simulink model "sadycos"  (R2024b)
settings: Solver=VariableStepAuto  StartTime=0.0  StopTime=60  RelTol=1e-3
undefined symbols (not defined in the file): BusTemplates, Parameters
settings Model: Creator=Friedrich Tuttas  LastModifiedBy=fn103921
settings DebuggingCC: AllowedUnitSystems=SI,SI (extended)
settings RTWCC: GPUComputeCapability=3.5

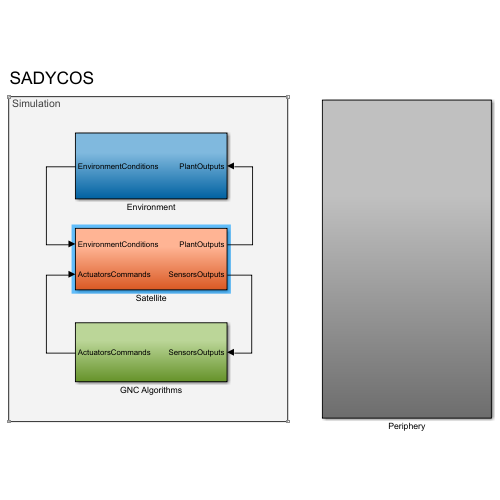
[thumbnail: Simulink's stored preview of the top-level diagram]
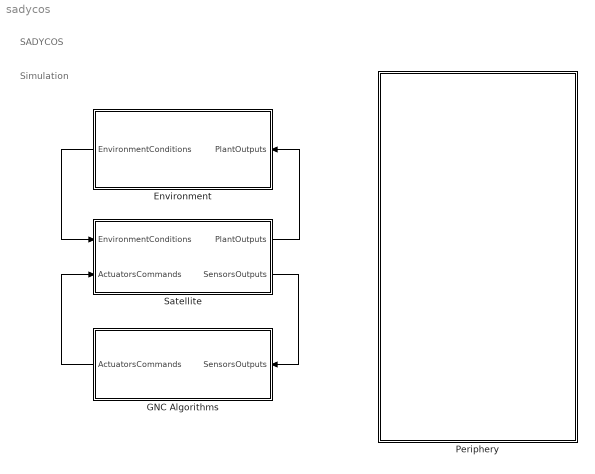
== system sadycos ==
  note: SADYCOS
  note: Simulation
  Environment : Subsystem
  GNC Algorithms : Subsystem
  Periphery : Subsystem
  Satellite : Subsystem
  wires:
  Satellite/1(PlantOutputs) -> Environment/1(PlantOutputs)
  Satellite/2(SensorsOutputs) -> GNC Algorithms/1(SensorsOutputs)
  GNC Algorithms/1(ActuatorsCommands) -> Satellite/2(ActuatorsCommands)
  Environment/1(EnvironmentConditions) -> Satellite/1(EnvironmentConditions)

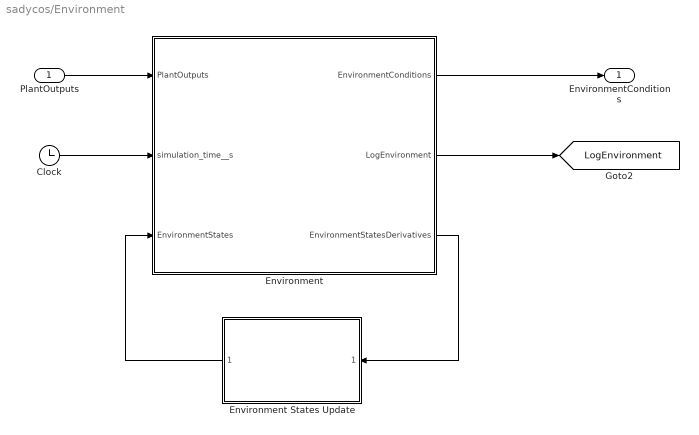
== system sadycos/Environment ==
  PlantOutputs : Inport
  Clock : Clock
  Environment : MATLAB Function  TreatAsAtomicUnit=on  SystemSampleTime=[0 0]
  Environment States Update : Subsystem  ReferencedSubsystem=states_update  states_type=Parameters.General.States.Type.Environment  bus=EnvironmentStates  BusTemplate=BusTemplates.EnvironmentStates  BusInitialValue=Parameters.General.States.InitialStates.Environment
  EnvironmentConditions : Outport
  tag scope: LogEnvironment=global
  wires:
  PlantOutputs/1 -> Environment/1(PlantOutputs)
  Clock/1 -> Environment/2(simulation_time__s)
  Environment/1(EnvironmentConditions) -> EnvironmentConditions/1
  Environment/3(EnvironmentStatesDerivatives) -> Environment States Update/1
  Environment/2(LogEnvironment) -> [LogEnvironment]
  Environment States Update/1 -> Environment/3(EnvironmentStates)

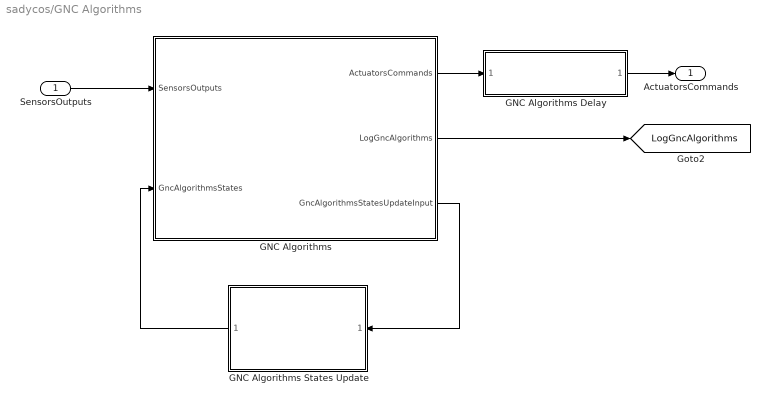
== system sadycos/GNC Algorithms ==
  SensorsOutputs : Inport
  GNC Algorithms : MATLAB Function  TreatAsAtomicUnit=on  SystemSampleTime=Parameters.General.SampleTimeParameters__s.GncAlgorithms
  GNC Algorithms Delay : Subsystem  ReferencedSubsystem=delay  delay_type=Parameters.General.Delays.Type.GncAlgorithms  delay_value=Parameters.General.Delays.Value.GncAlgorithms  bus=ActuatorsCommands  BusTemplate=BusTemplates.ActuatorsCommands  BusInitialValue=Parameters.General.Delays.InitialOutputs.GncAlgorithms
  GNC Algorithms States Update : Subsystem  ReferencedSubsystem=states_update  states_type=Parameters.General.States.Type.GncAlgorithms  bus=GncAlgorithmsStates  BusTemplate=BusTemplates.GncAlgorithmsStates  BusInitialValue=Parameters.General.States.InitialStates.GncAlgorithms
  ActuatorsCommands : Outport
  tag scope: LogGncAlgorithms=global
  wires:
  SensorsOutputs/1 -> GNC Algorithms/1(SensorsOutputs)
  GNC Algorithms States Update/1 -> GNC Algorithms/2(GncAlgorithmsStates)
  GNC Algorithms/3(GncAlgorithmsStatesUpdateInput) -> GNC Algorithms States Update/1
  GNC Algorithms/1(ActuatorsCommands) -> GNC Algorithms Delay/1
  GNC Algorithms Delay/1 -> ActuatorsCommands/1
  GNC Algorithms/2(LogGncAlgorithms) -> [LogGncAlgorithms]

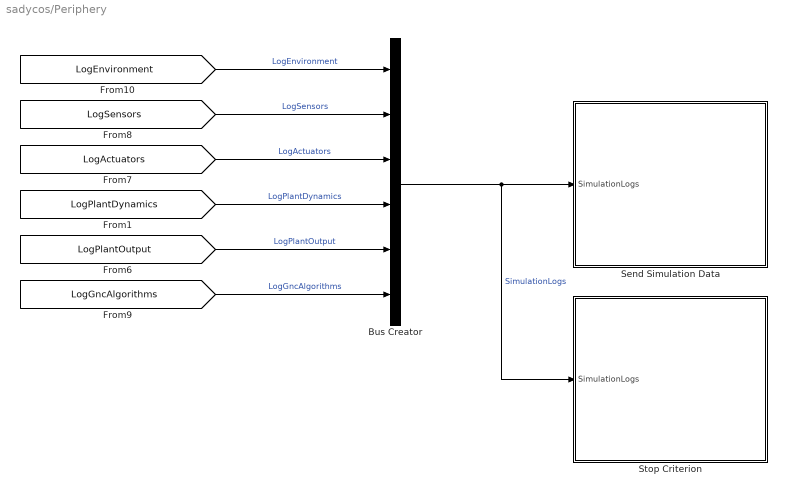
== system sadycos/Periphery ==
  Bus Creator : BusCreator  Inputs=6
  Send Simulation Data : Subsystem  Variant=on
  Stop Criterion : Subsystem  Variant=on
  wires:
  [LogEnvironment] -> Bus Creator/1  "LogEnvironment"
  [LogSensors] -> Bus Creator/2  "LogSensors"
  [LogActuators] -> Bus Creator/3  "LogActuators"
  [LogPlantDynamics] -> Bus Creator/4  "LogPlantDynamics"
  [LogGncAlgorithms] -> Bus Creator/6  "LogGncAlgorithms"
  Bus Creator/1 -> Stop Criterion/1(SimulationLogs), Send Simulation Data/1(SimulationLogs)  "SimulationLogs"
  [LogPlantOutput] -> Bus Creator/5  "LogPlantOutput"

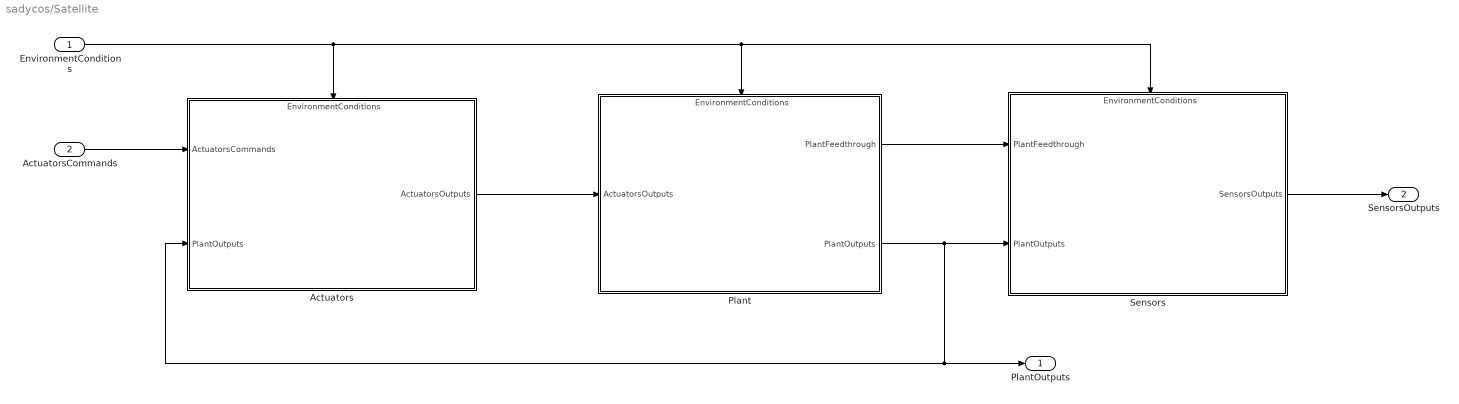
== system sadycos/Satellite ==
  EnvironmentConditions : Inport
  ActuatorsCommands : Inport  Port=2
  Actuators : Subsystem
      settings: PortSchema="{\"entries\":[{\"content\":{\"sides\":[{\"content\":{\"connectorIds\":[\"In1\",\"In2\"]},\"type\":\"ConnectorPlacement.EquallySpacedRectSide\",\"uuid\":\"84ab0471-c988-440c-b8b5-169cbd29501d\"},{\"content\":{\"connectorIds\":[\"Out1\"],\"side\":\"RIGHT\"},\"type\":\"ConnectorPlacement.EquallySpacedRectSide\",\"uuid\":\"27e08eb0-e385-4cd2-ab07-f71ebf995a80\"},{\"content\":{\"connectorIds\":[\"In3\"],\"side\":\"TOP\"},\"type\":\"ConnectorPlacement.EquallySpacedRectSide\",\"uuid\":\"cab321e1-33b2-485e-b5bf-fb44744ac506\"}]},\"type\":\"ConnectorPlacement.EquallySpacedConnector\",\"uuid\":\"5928dd13-f33e-440f-ae50-e37070d8560c\"}],\"packageUris\":[\"http://schema.mathworks.com/mf0/Connector/R2020b\"],\"version\":\"1.0\"}"
  Plant : Subsystem
      settings: PortSchema="{\"entries\":[{\"content\":{\"sides\":[{\"content\":{\"connectorIds\":[\"In1\"]},\"type\":\"ConnectorPlacement.EquallySpacedRectSide\",\"uuid\":\"699a6fa8-6c9c-46ad-a38d-56c4e347c077\"},{\"content\":{\"connectorIds\":[\"Out1\",\"Out2\"],\"side\":\"RIGHT\"},\"type\":\"ConnectorPlacement.EquallySpacedRectSide\",\"uuid\":\"694d06d3-80f5-4508-a5d9-bbea1f4beed1\"},{\"content\":{\"connectorIds\":[\"In2\"],\"side\":\"TOP\"},\"type\":\"ConnectorPlacement.EquallySpacedRectSide\",\"uuid\":\"e94fc242-ccf1-4a3f-a0a3-aabba68462ab\"}]},\"type\":\"ConnectorPlacement.EquallySpacedConnector\",\"uuid\":\"3ec82bb7-f16b-4cee-bf6e-85b229f26cd9\"}],\"packageUris\":[\"http://schema.mathworks.com/mf0/Connector/R2020b\"],\"version\":\"1.0\"}"
  Sensors : Subsystem
      settings: PortSchema="{\"entries\":[{\"content\":{\"sides\":[{\"content\":{\"connectorIds\":[\"In1\",\"In2\"]},\"type\":\"ConnectorPlacement.EquallySpacedRectSide\",\"uuid\":\"84ab0471-c988-440c-b8b5-169cbd29501d\"},{\"content\":{\"connectorIds\":[\"Out1\"],\"side\":\"RIGHT\"},\"type\":\"ConnectorPlacement.EquallySpacedRectSide\",\"uuid\":\"27e08eb0-e385-4cd2-ab07-f71ebf995a80\"},{\"content\":{\"connectorIds\":[\"In3\"],\"side\":\"TOP\"},\"type\":\"ConnectorPlacement.EquallySpacedRectSide\",\"uuid\":\"cab321e1-33b2-485e-b5bf-fb44744ac506\"}]},\"type\":\"ConnectorPlacement.EquallySpacedConnector\",\"uuid\":\"5928dd13-f33e-440f-ae50-e37070d8560c\"}],\"packageUris\":[\"http://schema.mathworks.com/mf0/Connector/R2020b\"],\"version\":\"1.0\"}"
  PlantOutputs : Outport
  SensorsOutputs : Outport  Port=2
  wires:
  EnvironmentConditions/1 -> Actuators/3(EnvironmentConditions), Plant/2(EnvironmentConditions), Sensors/3(EnvironmentConditions)
  Plant/2(PlantOutputs) -> PlantOutputs/1, Actuators/2(PlantOutputs), Sensors/2(PlantOutputs)
  Plant/1(PlantFeedthrough) -> Sensors/1(PlantFeedthrough)
  Sensors/1(SensorsOutputs) -> SensorsOutputs/1
  ActuatorsCommands/1 -> Actuators/1(ActuatorsCommands)
  Actuators/1(ActuatorsOutputs) -> Plant/1(ActuatorsOutputs)

== system sadycos/Periphery/Send Simulation Data ==
  note: 1) Add Subsystem or Model blocks as valid variant choices.
      | 2) You cannot connect blocks at this level. At simulation, connectivity is automatically
      | determined, based on the active variant and port name matching.
  SimulationLogs : Inport
  Off : Subsystem  VariantControl=~Parameters.General.enable_send_sim_data
  On : Subsystem  VariantControl=Parameters.General.enable_send_sim_data

== system sadycos/Periphery/Stop Criterion ==
  note: 1) Add Subsystem or Model blocks as valid variant choices.
      | 2) You cannot connect blocks at this level. At simulation, connectivity is automatically
      | determined, based on the active variant and port name matching.
  SimulationLogs : Inport
  Off : Subsystem  VariantControl=~Parameters.General.enable_stop_criterion
  On : Subsystem  VariantControl=Parameters.General.enable_stop_criterion

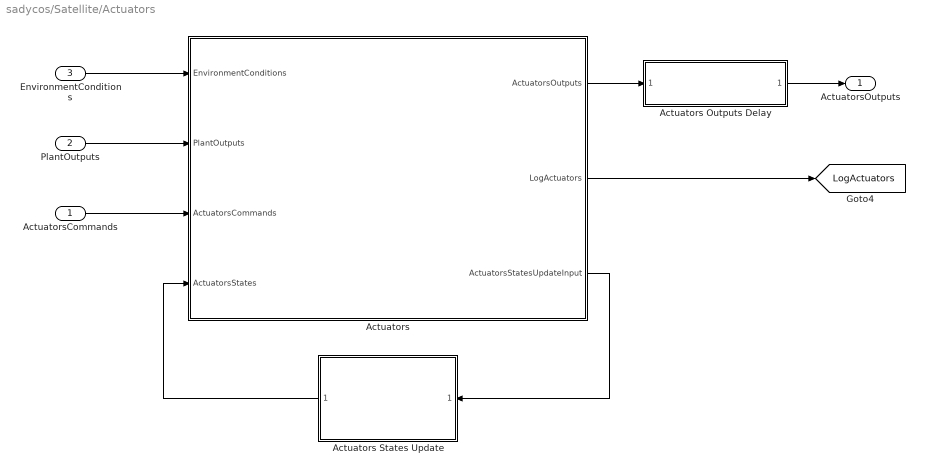
== system sadycos/Satellite/Actuators ==
  ActuatorsCommands : Inport
  PlantOutputs : Inport  Port=2
  EnvironmentConditions : Inport  Port=3
  Actuators : MATLAB Function  TreatAsAtomicUnit=on  SystemSampleTime=Parameters.General.SampleTimeParameters__s.Sensors
  Actuators States Update : Subsystem  ReferencedSubsystem=states_update  states_type=Parameters.General.States.Type.Actuators  bus=ActuatorsStates  BusTemplate=BusTemplates.ActuatorsStates  BusInitialValue=Parameters.General.States.InitialStates.Actuators
  Actuators Outputs Delay : Subsystem  ReferencedSubsystem=delay  delay_type=Parameters.General.Delays.Type.Actuators  delay_value=Parameters.General.Delays.Value.Actuators  bus=ActuatorsOutputs  BusTemplate=BusTemplates.ActuatorsOutputs  BusInitialValue=Parameters.General.Delays.InitialOutputs.Actuators
  ActuatorsOutputs : Outport
  tag scope: LogActuators=global
  wires:
  ActuatorsCommands/1 -> Actuators/3(ActuatorsCommands)
  Actuators States Update/1 -> Actuators/4(ActuatorsStates)
  EnvironmentConditions/1 -> Actuators/1(EnvironmentConditions)
  PlantOutputs/1 -> Actuators/2(PlantOutputs)
  Actuators Outputs Delay/1 -> ActuatorsOutputs/1
  Actuators/3(ActuatorsStatesUpdateInput) -> Actuators States Update/1
  Actuators/2(LogActuators) -> [LogActuators]
  Actuators/1(ActuatorsOutputs) -> Actuators Outputs Delay/1

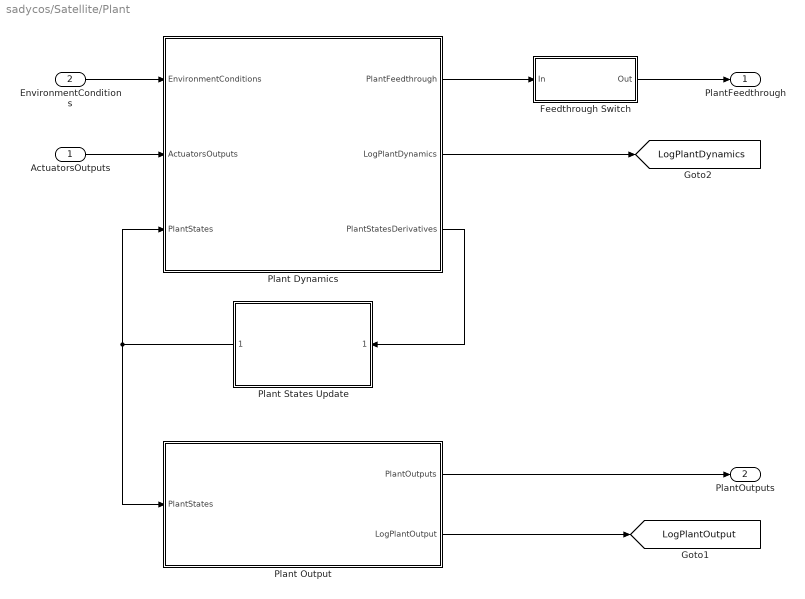
== system sadycos/Satellite/Plant ==
  ActuatorsOutputs : Inport
  EnvironmentConditions : Inport  Port=2
  Feedthrough Switch : Subsystem  Variant=on
  Plant States Update : Subsystem  ReferencedSubsystem=states_update  states_type="\"continuous\""  bus=PlantStates  BusTemplate=BusTemplates.PlantStates  BusInitialValue=Parameters.General.States.InitialStates.Plant
  Plant Dynamics : MATLAB Function  TreatAsAtomicUnit=on  SystemSampleTime=[0 0]
  Plant Output : MATLAB Function  TreatAsAtomicUnit=on  SystemSampleTime=[0 0]
  PlantFeedthrough : Outport
  PlantOutputs : Outport  Port=2
  tag scope: LogPlantDynamics=global, LogPlantOutput=global
  wires:
  Plant States Update/1 -> Plant Output/1(PlantStates), Plant Dynamics/3(PlantStates)
  Plant Dynamics/1(PlantFeedthrough) -> Feedthrough Switch/1(In)
  Plant Output/1(PlantOutputs) -> PlantOutputs/1
  ActuatorsOutputs/1 -> Plant Dynamics/2(ActuatorsOutputs)
  EnvironmentConditions/1 -> Plant Dynamics/1(EnvironmentConditions)
  Plant Dynamics/3(PlantStatesDerivatives) -> Plant States Update/1
  Plant Dynamics/2(LogPlantDynamics) -> [LogPlantDynamics]
  Plant Output/2(LogPlantOutput) -> [LogPlantOutput]
  Feedthrough Switch/1(Out) -> PlantFeedthrough/1

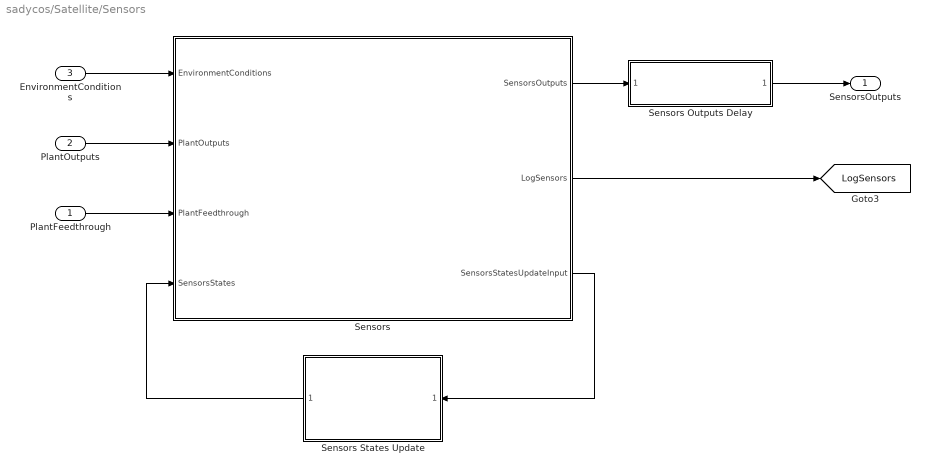
== system sadycos/Satellite/Sensors ==
  PlantFeedthrough : Inport
  PlantOutputs : Inport  Port=2
  EnvironmentConditions : Inport  Port=3
  Sensors : MATLAB Function  TreatAsAtomicUnit=on  SystemSampleTime=Parameters.General.SampleTimeParameters__s.Sensors
  Sensors States Update : Subsystem  ReferencedSubsystem=states_update  states_type=Parameters.General.States.Type.Sensors  bus=EnvironmentStates  BusTemplate=BusTemplates.EnvironmentStates  BusInitialValue=Parameters.General.States.InitialStates.Sensors
  Sensors Outputs Delay : Subsystem  ReferencedSubsystem=delay  delay_type=Parameters.General.Delays.Type.Sensors  delay_value=Parameters.General.Delays.Value.Sensors  bus=SensorsOutputs  BusTemplate=BusTemplates.SensorsOutputs  BusInitialValue=Parameters.General.Delays.InitialOutputs.Sensors
  SensorsOutputs : Outport
  tag scope: LogSensors=global
  wires:
  PlantOutputs/1 -> Sensors/2(PlantOutputs)
  Sensors/2(LogSensors) -> [LogSensors]
  Sensors Outputs Delay/1 -> SensorsOutputs/1
  Sensors/3(SensorsStatesUpdateInput) -> Sensors States Update/1
  PlantFeedthrough/1 -> Sensors/3(PlantFeedthrough)
  Sensors/1(SensorsOutputs) -> Sensors Outputs Delay/1
  EnvironmentConditions/1 -> Sensors/1(EnvironmentConditions)
  Sensors States Update/1 -> Sensors/4(SensorsStates)

== system sadycos/Periphery/Send Simulation Data/Off ==
  SimulationLogs : Inport
  Terminator : Terminator
  wires:
  SimulationLogs/1 -> Terminator/1

== system sadycos/Periphery/Send Simulation Data/On ==
  SimulationLogs : Inport
  UDP Output : Subsystem
  wires:
  SimulationLogs/1 -> UDP Output/1(SimulationLogs)

== system sadycos/Periphery/Stop Criterion/Off ==
  SimulationLogs : Inport
  Terminator : Terminator
  wires:
  SimulationLogs/1 -> Terminator/1

== system sadycos/Periphery/Stop Criterion/On ==
  SimulationLogs : Inport
  Stop Criterion : Subsystem
  wires:
  SimulationLogs/1 -> Stop Criterion/1(SimulationLogs)

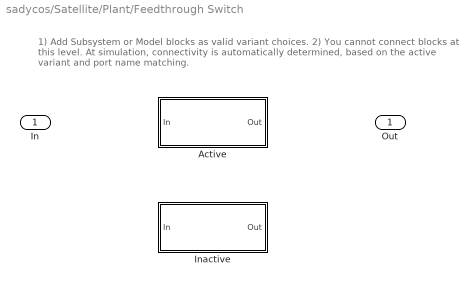
== system sadycos/Satellite/Plant/Feedthrough Switch ==
  note: 1) Add Subsystem or Model blocks as valid variant choices.
      | 2) You cannot connect blocks at this level. At simulation, connectivity is automatically
      | determined, based on the active variant and port name matching.
  In : Inport
  Active : Subsystem  VariantControl=Parameters.General.enable_plant_feedthrough
  Inactive : Subsystem  VariantControl=~Parameters.General.enable_plant_feedthrough
  Out : Outport

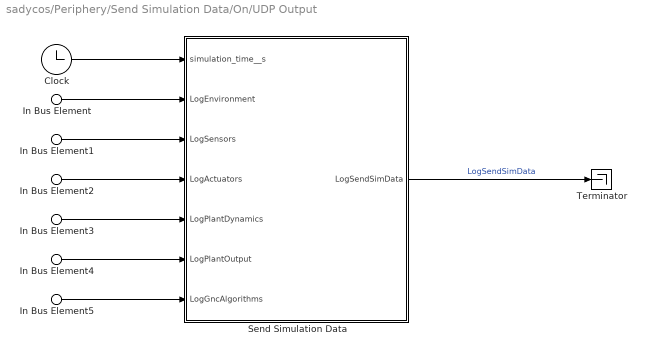
== system sadycos/Periphery/Send Simulation Data/On/UDP Output ==
  In Bus Element : Inport  PortName=SimulationLogs  Element=LogEnvironment
  In Bus Element1 : Inport  PortName=SimulationLogs  Element=LogSensors
  In Bus Element2 : Inport  PortName=SimulationLogs  Element=LogActuators
  In Bus Element3 : Inport  PortName=SimulationLogs  Element=LogPlantDynamics
  In Bus Element4 : Inport  PortName=SimulationLogs  Element=LogPlantOutput
  In Bus Element5 : Inport  PortName=SimulationLogs  Element=LogGncAlgorithms
  Clock : Clock
  Send Simulation Data : MATLAB Function  TreatAsAtomicUnit=on  SystemSampleTime=0
  Terminator : Terminator
  wires:
  Clock/1 -> Send Simulation Data/1(simulation_time__s)
  Send Simulation Data/1(LogSendSimData) -> Terminator/1  "LogSendSimData"
  In Bus Element/1 -> Send Simulation Data/2(LogEnvironment)
  In Bus Element1/1 -> Send Simulation Data/3(LogSensors)
  In Bus Element2/1 -> Send Simulation Data/4(LogActuators)
  In Bus Element3/1 -> Send Simulation Data/5(LogPlantDynamics)
  In Bus Element4/1 -> Send Simulation Data/6(LogPlantOutput)
  In Bus Element5/1 -> Send Simulation Data/7(LogGncAlgorithms)

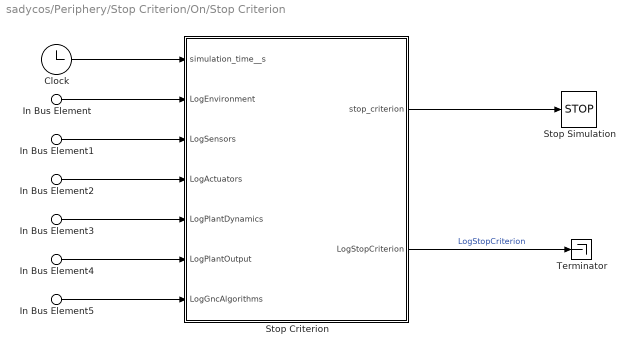
== system sadycos/Periphery/Stop Criterion/On/Stop Criterion ==
  In Bus Element : Inport  PortName=SimulationLogs  Element=LogEnvironment
  In Bus Element1 : Inport  PortName=SimulationLogs  Element=LogSensors
  In Bus Element2 : Inport  PortName=SimulationLogs  Element=LogActuators
  In Bus Element3 : Inport  PortName=SimulationLogs  Element=LogPlantDynamics
  In Bus Element4 : Inport  PortName=SimulationLogs  Element=LogPlantOutput
  In Bus Element5 : Inport  PortName=SimulationLogs  Element=LogGncAlgorithms
  Clock : Clock
  Stop Criterion : MATLAB Function  TreatAsAtomicUnit=on  SystemSampleTime=0
  Stop Simulation : Stop
  Terminator : Terminator
  wires:
  In Bus Element5/1 -> Stop Criterion/7(LogGncAlgorithms)
  In Bus Element4/1 -> Stop Criterion/6(LogPlantOutput)
  In Bus Element3/1 -> Stop Criterion/5(LogPlantDynamics)
  In Bus Element2/1 -> Stop Criterion/4(LogActuators)
  In Bus Element1/1 -> Stop Criterion/3(LogSensors)
  In Bus Element/1 -> Stop Criterion/2(LogEnvironment)
  Stop Criterion/2(LogStopCriterion) -> Terminator/1  "LogStopCriterion"
  Clock/1 -> Stop Criterion/1(simulation_time__s)
  Stop Criterion/1(stop_criterion) -> Stop Simulation/1

== system sadycos/Satellite/Plant/Feedthrough Switch/Active ==
  In : Inport
  Out : Outport
  wires:
  In/1 -> Out/1

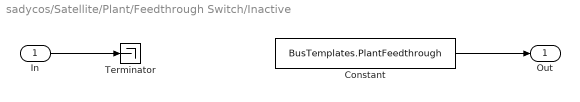
== system sadycos/Satellite/Plant/Feedthrough Switch/Inactive ==
  In : Inport
  Constant : Constant  Value=BusTemplates.PlantFeedthrough  OutDataTypeStr=Bus: PlantFeedthrough
  Terminator : Terminator
  Out : Outport
  wires:
  In/1 -> Terminator/1
  Constant/1 -> Out/1

== matlab function sadycos/Satellite/Plant/Plant Dynamics ==
  data: PlantFeedthrough output Bus: PlantFeedthrough; LogPlantDynamics output Bus: LogPlantDynamics; EnvironmentConditions input; PlantStatesDerivatives output Bus: PlantStates; ActuatorsOutputs input; PlantStates input; Parameters parameter; BusTemplates parameter
function [PlantFeedthrough, ...
            LogPlantDynamics, ...    
            PlantStatesDerivatives] ...
            = PlantDynamics(EnvironmentConditions, ...
                            ActuatorsOutputs, ...
                            PlantStates, ...
                            Parameters, ...
                            BusTemplates)

%% Parameters Abbreviations
ParametersPlant = Parameters.Plant;

%% Initialize Bus Outputs
PlantFeedthrough = BusTemplates.PlantFeedthrough;
LogPlantDynamics = BusTemplates.LogPlantDynamics;
PlantStatesDerivatives = BusTemplates.PlantStates;

%% Call Function
[PlantFeedthrough, ...
    LogPlantDynamics, ...    
    PlantStatesDerivatives] ...
    = SimulinkInterfaces.plantDynamics(PlantFeedthrough, ...
                                        LogPlantDynamics, ...
                                        PlantStatesDerivatives, ...
                                        EnvironmentConditions, ...
                                        ActuatorsOutputs, ...
                                        PlantStates, ...
                                        ParametersPlant);

end

== matlab function sadycos/Periphery/Stop Criterion/On/Stop Criterion/Stop Criterion ==
  data: simulation_time__s input; LogEnvironment input; LogSensors input; LogActuators input; LogPlantDynamics input; LogPlantOutput input; LogGncAlgorithms input; Parameters parameter; stop_criterion output; LogStopCriterion output Bus: LogStopCriterion; BusTemplates parameter
function [stop_criterion, LogStopCriterion] = StopCriterion(simulation_time__s, ...
                                                            LogEnvironment, ...
                                                            LogSensors, ...
                                                            LogActuators, ...
                                                            LogPlantDynamics, ...
                                                            LogPlantOutput,...
                                                            LogGncAlgorithms, ...
                                                            Parameters, ...
                                                            BusTemplates)
%% Initialize Bus Outputs
LogStopCriterion = BusTemplates.LogStopCriterion;

%% Call Function
[stop_criterion, LogStopCriterion] ...
    = SimulinkInterfaces.stopCriterion(LogStopCriterion, ...
                                        simulation_time__s, ...
                                        LogEnvironment, ...
                                        LogSensors, ...
                                        LogActuators, ...
                                        LogPlantDynamics, ...
                                        LogPlantOutput,...
                                        LogGncAlgorithms, ...
                                        Parameters);

== matlab function sadycos/Satellite/Plant/Plant Output ==
  data: PlantOutputs output Bus: PlantOutputs; PlantStates input; Parameters parameter; BusTemplates parameter; LogPlantOutput output Bus: LogPlantOutput
function [PlantOutputs, LogPlantOutput] = PlantOutput(PlantStates, Parameters, BusTemplates)

%% Parameters Abbreviations
ParametersPlant = Parameters.Plant;

%% Initialize Bus Outputs
PlantOutputs = BusTemplates.PlantOutputs;
LogPlantOutput = BusTemplates.LogPlantOutput;

%% Call Function
[PlantOutputs, LogPlantOutput] ...
    = SimulinkInterfaces.plantOutput(PlantOutputs, ...
                                    LogPlantOutput, ...
                                    PlantStates, ...
                                    ParametersPlant);

== matlab function sadycos/Periphery/Send Simulation Data/On/UDP Output/Send Simulation Data ==
  data: simulation_time__s input; LogEnvironment input; LogSensors input; LogActuators input; LogPlantDynamics input; LogPlantOutput input; LogGncAlgorithms input; Parameters parameter; LogSendSimData output Bus: LogSendSimData; BusTemplates parameter
function LogSendSimData  = SendSimData(simulation_time__s, ...
                                                            LogEnvironment, ...
                                                            LogSensors, ...
                                                            LogActuators, ...
                                                            LogPlantDynamics, ...
                                                            LogPlantOutput,...
                                                            LogGncAlgorithms, ...
                                                            Parameters, ...
                                                            BusTemplates)
%% Initialize Bus Outputs
LogSendSimData = BusTemplates.LogSendSimData;

%% Call Function
[udp_data_vector, LogSendSimData] ...
    = SimulinkInterfaces.sendSimData(LogSendSimData, ...
                                        simulation_time__s, ...
                                        LogEnvironment, ...
                                        LogSensors, ...
                                        LogActuators, ...
                                        LogPlantDynamics, ...
                                        LogPlantOutput,...
                                        LogGncAlgorithms, ...
                                        Parameters);

== matlab function sadycos/Satellite/Sensors/Sensors ==
  data: EnvironmentConditions input; PlantOutputs input; PlantFeedthrough input; SensorsOutputs output Bus: SensorsOutputs; LogSensors output Bus: LogSensors; SensorsStates input; SensorsStatesUpdateInput output Bus: SensorsStates; Parameters parameter; BusTemplates parameter
function [SensorsOutputs, ...
            LogSensors, ...
            SensorsStatesUpdateInput] ...
            = Sensors(EnvironmentConditions, ...
                        PlantOutputs, ...
                        PlantFeedthrough, ...
                        SensorsStates, ...
                        Parameters, ...
                        BusTemplates)

%% Parameters Abbreviations
ParametersSensors = Parameters.Sensors;

%% Initialize Bus Outputs
SensorsOutputs = BusTemplates.SensorsOutputs;
LogSensors = BusTemplates.LogSensors;
SensorsStatesUpdateInput = BusTemplates.SensorsStates;

%% Call Function
[SensorsOutputs, ...
    LogSensors, ...
    SensorsStatesUpdateInput] ...
    = SimulinkInterfaces.sensors(SensorsOutputs, ...
                                    LogSensors, ...
                                    SensorsStatesUpdateInput, ...
                                    EnvironmentConditions, ...
                                    PlantOutputs, ...
                                    PlantFeedthrough, ...
                                    SensorsStates, ...
                                    ParametersSensors);

end

== matlab function sadycos/Environment/Environment ==
  data: PlantOutputs input; EnvironmentConditions output Bus: EnvironmentConditions; LogEnvironment output Bus: LogEnvironment; simulation_time__s input; EnvironmentStates input; EnvironmentStatesDerivatives output Bus: EnvironmentStates; Parameters parameter; BusTemplates parameter
function [EnvironmentConditions, ...
            LogEnvironment, ...
            EnvironmentStatesDerivatives] ...
            = Environment(PlantOutputs, ...
                            simulation_time__s, ...
                            EnvironmentStates, ...
                            Parameters, ...
                            BusTemplates)

%% Parameters Abbreviations
ParametersEnvironment = Parameters.Environment;

%% Initialize Bus Outputs
EnvironmentConditions = BusTemplates.EnvironmentConditions;
LogEnvironment = BusTemplates.LogEnvironment;
EnvironmentStatesDerivatives = BusTemplates.EnvironmentStates;

%% Call Function
[EnvironmentConditions, ...
    LogEnvironment, ...
    EnvironmentStatesDerivatives] ...
    = SimulinkInterfaces.environment(EnvironmentConditions, ...
                                        LogEnvironment, ...
                                        EnvironmentStatesDerivatives, ...
                                        PlantOutputs, ...
                                        simulation_time__s, ...
                                        EnvironmentStates, ...
                                        ParametersEnvironment);
end

== matlab function sadycos/GNC Algorithms/GNC Algorithms ==
  data: SensorsOutputs input; ActuatorsCommands output Bus: ActuatorsCommands; GncAlgorithmsStates input; LogGncAlgorithms output Bus: LogGncAlgorithms; Parameters parameter; GncAlgorithmsStatesUpdateInput output Bus: GncAlgorithmsStates; BusTemplates parameter
function [ActuatorsCommands, ...
            LogGncAlgorithms, ...
            GncAlgorithmsStatesUpdateInput] ...
            = GncAlgorithms(SensorsOutputs,...
                            GncAlgorithmsStates, ...
                            Parameters, ...
                            BusTemplates)

%% Parameters Abbreviations
ParametersGncAlgorithms = Parameters.GncAlgorithms;

%% Initialize Bus Outputs
ActuatorsCommands = BusTemplates.ActuatorsCommands;
LogGncAlgorithms = BusTemplates.LogGncAlgorithms;
GncAlgorithmsStatesUpdateInput = BusTemplates.GncAlgorithmsStates;

%% Call Function
[ActuatorsCommands, ...
    LogGncAlgorithms, ...
    GncAlgorithmsStatesUpdateInput] ...
    = SimulinkInterfaces.gncAlgorithms(ActuatorsCommands, ...
                                        LogGncAlgorithms, ...
                                        GncAlgorithmsStatesUpdateInput, ...
                                        SensorsOutputs, ...
                                        GncAlgorithmsStates, ...
                                        ParametersGncAlgorithms);


end

== matlab function sadycos/Satellite/Actuators/Actuators ==
  data: ActuatorsOutputs output Bus: ActuatorsOutputs; LogActuators output Bus: LogActuators; EnvironmentConditions input; PlantOutputs input; ActuatorsCommands input; ActuatorsStates input; ActuatorsStatesUpdateInput output Bus: ActuatorsStates; Parameters parameter; BusTemplates parameter
function [ActuatorsOutputs, ...
            LogActuators, ...
            ActuatorsStatesUpdateInput] ...
            = Actuators(EnvironmentConditions, ...
                        PlantOutputs, ...
                        ActuatorsCommands, ...
                        ActuatorsStates, ...
                        Parameters, ...
                        BusTemplates)

%% Parameters Abbreviations
ParametersActuators = Parameters.Actuators;

%% Initialize Bus Outputs
ActuatorsOutputs = BusTemplates.ActuatorsOutputs;
LogActuators = BusTemplates.LogActuators;
ActuatorsStatesUpdateInput = BusTemplates.ActuatorsStates;

%% Call Function
[ActuatorsOutputs,...
    LogActuators, ...
    ActuatorsStatesUpdateInput] ...
    = SimulinkInterfaces.actuators(ActuatorsOutputs, ...
                                    LogActuators, ...
                                    ActuatorsStatesUpdateInput, ...
                                    EnvironmentConditions, ...
                                    PlantOutputs, ...
                                    ActuatorsCommands, ...
                                    ActuatorsStates, ...
                                    ParametersActuators);

end
